simulink model "modeloSimulinkShinskey"  (R2019a)
settings: Solver=VariableStepAuto  StartTime=0.0  StopTime=2000  RelTol=1e-3
libraries: dspsrcs4 x1
settings Model: Creator=Laura  LastModifiedBy=Laura

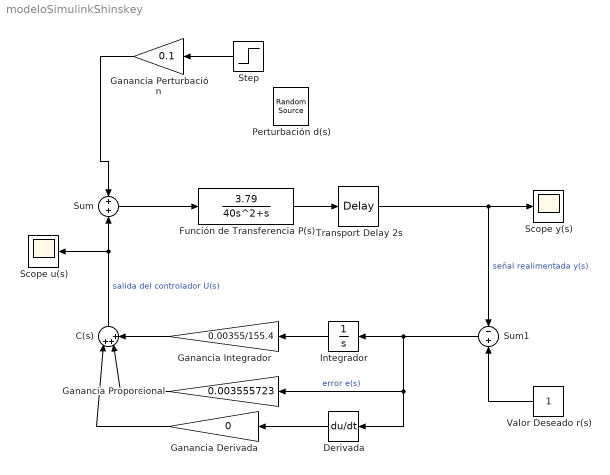
== system modeloSimulinkShinskey ==
  " C(s)" : Sum  Inputs=|+++
  Derivada : Derivative
  Función de Transferencia P(s) : TransferFcn  Numerator=[3.79]  Denominator=[40 1 0]
  Ganancia Derivada : Gain  Gain=0
  Ganancia Integrador : Gain  Gain=0.00355/155.4
  Ganancia Perturbación : Gain  Gain=0.1
  Ganancia Proporcional : Gain  Gain=0.003555723
  Integrador : Integrator
  "Perturbación d(s) " : dspsrcs4/Random Source  SrcType=Uniform  NormMethod=Ziggurat  CltLength=12  MinVal=0  MaxVal=1  MeanVal=0  VarVal=1  RepMode=Not repeatable  rawSeed=1  IsInherit=off  SampMode=Discrete  SampTime=1  SampFrame=1  DataType=Double  OutComplex=Real  OutputFrames=off
  Scope u(s) : Scope
  Scope y(s) : Scope
  Step : Step  Time=1000  SampleTime=0
  Sum : Sum
  Sum1 : Sum  Inputs=-+
  Transport Delay 2s : TransportDelay  DelayTime=2
  Valor Deseado r(s) : Constant
  wires:
  Ganancia Perturbación/1 -> Sum/1
  Valor Deseado r(s)/1 -> Sum1/2
  Sum1/1 -> Ganancia Proporcional/1, Derivada/1, Integrador/1  "error e(s)"
  Integrador/1 -> Ganancia Integrador/1
  Derivada/1 -> Ganancia Derivada/1
  Ganancia Integrador/1 -> " C(s)"/3
  Ganancia Proporcional/1 -> " C(s)"/2
  Ganancia Derivada/1 -> " C(s)"/1
  " C(s)"/1 -> Scope u(s)/1, Sum/2  "salida del controlador U(s)"
  Sum/1 -> Función de Transferencia P(s)/1
  Transport Delay 2s/1 -> Scope y(s)/1, Sum1/1  "señal realimentada y(s)"
  Función de Transferencia P(s)/1 -> Transport Delay 2s/1
  Step/1 -> Ganancia Perturbación/1
